simulink model "audio_sine_notch"  (R2018b)
settings: Solver=VariableStepAuto  StartTime=0.0  StopTime=10.0  RelTol=1e-3
undefined symbols (not defined in the file or in its folder): dfilt
libraries: dspsnks4 x1, dsparch4 x1, dspvision x1
settings Model: Creator=Jason  LastModifiedBy=Jason
settings SFSimCC: SimUseLocalCustomCode=off
settings RTWCC: RTWUseLocalCustomCode=off
settings CodeAppCC: StateflowObjectComments=on

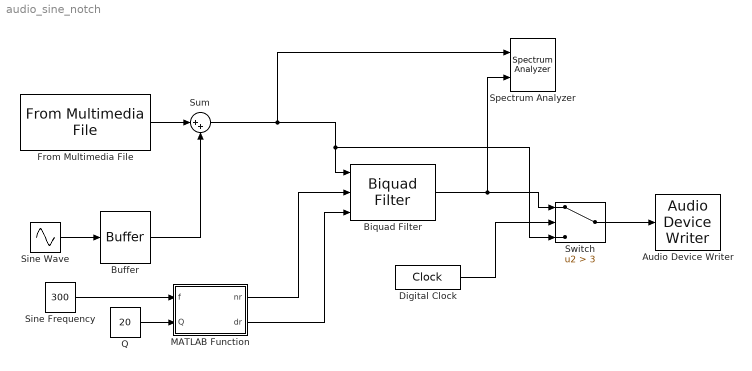
== system audio_sine_notch ==
  Audio Device Writer : dspsnks4/Audio Device Writer  Driver=DirectSound  Device=Default  InheritSampleRate=off  SampleRate=44100  BitDepth=16-bit integer  BufferSize=4096  NumBuffers=10  DefaultOutputChannelMapping=on  OutputChannelMapping=1:2  OutputNumUnderrunSamples=off  DriverIdx=1  DeviceWarnFlag=''
  Biquad Filter : dsparch4/Biquad Filter  FilterSource=Input port(s)  CoeffSource=Specify via dialog  FilterObject=dfilt.df2tsos([1 0.3 0.4],[1 0.1 0.2])  IIRFiltStruct=Direct form II transposed  BiQuadCoeffs=[1 0.3 0.4 1 0.1 0.2]  ScaleValues=1  IC=0  ICnum=0  ICden=0  a0Flag=Warning  optimizeScaleValues=on  ScaleValueMode=Assume all are unity and optimize  InputProcessing=Columns as channels (frame based)  roundingMode=Floor  overflowMode=off  scaleValueFracLength=14  denProdOutputFracLength=30  denAccumFracLength=30  secondMemoryFracLength=15
      settings: SourceProductName=DSP System Toolbox
  Buffer : Buffer  N=1024  OutputFrames=off
  Digital Clock : DigitalClock  SampleTime=1024/44100
  From Multimedia File : dspvision/From Multimedia File  inputFilename=C:\Users\Jason\Desktop\Lab2\guitar1.wav  loop=on  numPlays=inf  outputStreams=Audio only  videoDataType=single  audioDataType=double  inheritSampleTime=on  userDefinedSampleTime=1/30  noAudioOutput=off  isIntensityVideo=off  fourcc=RGB  colorVideoFormat=Separate color signals  outputEOF=off  dataOrg=Column-major  audioFrameSize=1024  computeAudioFrameSize=off  outSamplingMode=Sample based
      settings: SourceProductBaseCode=VP
  MATLAB Function : MATLAB Function  TreatAsAtomicUnit=on
  Q : Constant  Value=20
  Sine Frequency : Constant  Value=300
  Sine Wave : Sin  SineType=Sample based  Amplitude=0.5  Samples=44100/300  SampleTime=1/44100
  Spectrum Analyzer : SpectrumAnalyzer  NumInputPorts=2
  Sum : Sum  Inputs=|++
  Switch : Switch  Criteria=u2 > Threshold  Threshold=3
  wires:
  Sine Wave/1 -> Buffer/1
  From Multimedia File/1 -> Sum/1
  Buffer/1 -> Sum/2
  Sum/1 -> Spectrum Analyzer/1, Switch/3, Biquad Filter/1
  Q/1 -> MATLAB Function/2(Q)
  Sine Frequency/1 -> MATLAB Function/1(f)
  MATLAB Function/1(nr) -> Biquad Filter/2
  MATLAB Function/2(dr) -> Biquad Filter/3
  Digital Clock/1 -> Switch/2
  Biquad Filter/1 -> Spectrum Analyzer/2, Switch/1
  Switch/1 -> Audio Device Writer/1

== matlab function audio_sine_notch/MATLAB Function ==
  data: f input; nr output; Q input; dr output
function [nr, dr] = iirnotchS(f,Q)
%#codegen
lfo = f;
Fs = 44100;
Wo = (2*lfo/Fs)*pi;
BW = (2*lfo/Fs/Q)*pi;
Ab = 3;
Gb = 10^(-Ab/20);
beta = (sqrt(1-Gb.^2)/Gb)*tan(BW/2);
gain = 1/(1+beta);
b = gain*[1 -2*cos(Wo) 1];
a = [1 -2*gain*cos(Wo) (2*gain-1)];
dr = a(2:end)';
nr = b';
end
